simulink model "KV_testModel"  (R2018b)
settings: Solver=VariableStepAuto  StartTime=0.0  StopTime=10.0  RelTol=1e-3
undefined symbols (not defined in the file or in its folder): Ri_o, ul, Vi_o
libraries: nodeSpringDamperForce_ul x1
settings Model: Creator=asiddiq2  LastModifiedBy=asiddiq2

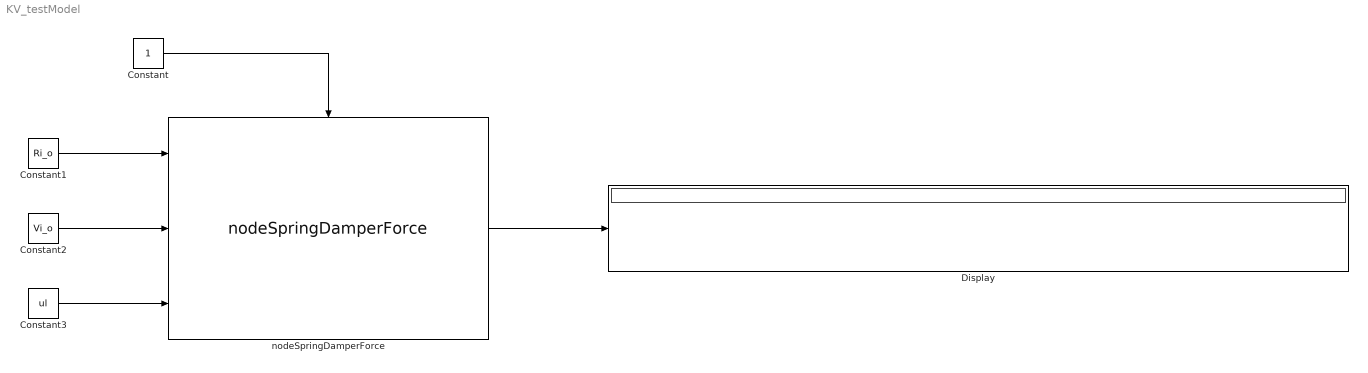
== system KV_testModel ==
  Constant : Constant
  Constant1 : Constant  Value=Ri_o
  Constant2 : Constant  Value=Vi_o  VectorParams1D=off
  Constant3 : Constant  Value=ul
  Display : Display
  nodeSpringDamperForce : nodeSpringDamperForce_ul/nodeSpringDamperForce  mass=mass  zeta=tdamp  diameter=tet_dia  youngsMod=tet_youngs
  wires:
  Constant/1 -> nodeSpringDamperForce/Enable
  Constant1/1 -> nodeSpringDamperForce/1
  Constant2/1 -> nodeSpringDamperForce/2
  Constant3/1 -> nodeSpringDamperForce/3
  nodeSpringDamperForce/1 -> Display/1
